simulink model "bicycle_drift_model_r_Ux_Uy"  (R2016a)
settings: Solver=VariableStepAuto  StartTime=0.0  StopTime=20  MaxStep=5e-2  RelTol=1e-3
values from neighbouring files (symbols this model uses):
  a = 0.1329    [dynamics.m]    (also in setup.m; tire_test.m = 0.11372)
  b = 0.1221    [dynamics.m]    (also in setup.m; tire_test.m = 0.14328)
  C_alpha = 120000    [dynamics.m]    (also in setup.m = 1200; tire_test.m = 197)
  initial_states_Uxy = [0.0 2 0]    [setup.m]
  Iz = 0.020899525    [dynamics.m]    (also in setup.m; tire_test.m = 0.025)
  L = 0.255    [dynamics.m]    (also in setup.m; tire_test.m = 0.257; veh_object2.m = obj_length)
  m = 2.622    [dynamics.m]    (also in setup.m; tire_test.m = 2.35)
  mu = 0.37    [dynamics.m]    (also in setup.m; tire_test.m = 1.31)
undefined symbols (not defined in the file): animation_update_interval, datetime, enable_CG_trace, enable_rearAxle_trace, plotAxisLimitMode, plotAxisLimits, save_anim_frames, vehicle_length, vehicle_width
libraries: vrlib x1, simulink x1
settings Model: Creator=Cyrus  LastModifiedBy=Cyrus

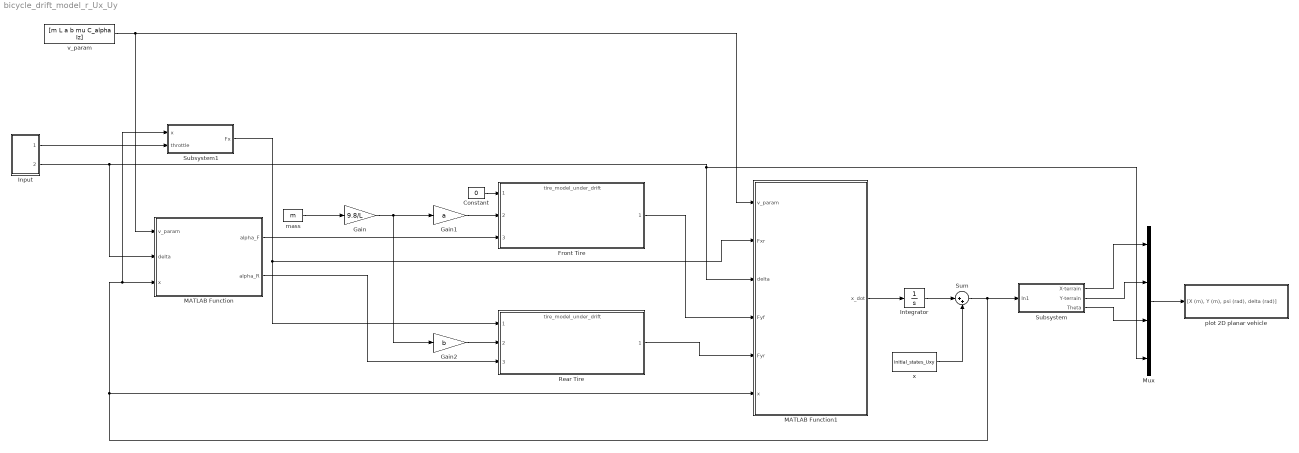
== system bicycle_drift_model_r_Ux_Uy ==
  Constant : Constant  Value=0
  Front Tire : ModelReference  ModelNameDialog=tire_model_under_drift.slx  SimulationMode=Normal  ModelReferenceVersion=1.36
  Gain : Gain  Gain=9.8/L
  Gain1 : Gain  Gain=a
  Gain2 : Gain  Gain=b
  Input : Subsystem
  Integrator : Integrator
  MATLAB Function : MATLAB Function  TreatAsAtomicUnit=on
  MATLAB Function1 : MATLAB Function  TreatAsAtomicUnit=on
  Mux : Mux
  Rear Tire : ModelReference  ModelNameDialog=tire_model_under_drift.slx  SimulationMode=Normal  ModelReferenceVersion=1.36
  Subsystem : Subsystem
  Subsystem1 : Subsystem
  Sum : Sum  Inputs=|++
  mass : Constant  Value=m
  plot 2D planar vehicle : Subsystem  mask(6DoF Animation){axisMode=plotAxisLimitMode, ax=plotAxisLimits, Ts=animation_update_interval, enable_CG_trace=enable_CG_trace, enable_rearAxle_trace=enable_rearAxle_trace, save_anim_frames=save_anim_frames, anim_frame_name_str=char(datetime('now','Format','yyyy-MM-dd_HH_mm_ss')), L=vehicle_length, W=vehicle_width}
      mask prompts: axisMode "Axis Mode (0->auto, 1->fixed, BOTH use Axes Limits below)"; ax "Axes limits [xmin xmax ymin ymax] (m):"; Ts "Time interval between updates (s):"; enable_CG_trace "Enable vehicle CG trace? (0/1)"; enable_rearAxle_trace "Enable rear axle trace? (0/1)"; save_anim_frames "Save animaton frames? (0/1)"; anim_frame_name_str "Animation sequence name (if save frames==1)"; L "Vehicle length (m)"; W "Vehicle width (m)"
      mask help:
      | Create a 2D animated view of a steering vehicle model with tires.
      |
      | Marc Compere
      | CompereM@saic.com
      | created : 22 August 2002
      | modified: 28 Dec 2015
      mask init:
      | Config.axisMode=axisMode;
      | Config.ax=ax;
      | Config.Ts=Ts;
      | Config.enable_CG_trace=enable_CG_trace;
      | Config.enable_rearAxle_trace=enable_rearAxle_trace;
      | Config.save_anim_frames=save_anim_frames;
      | Config.anim_frame_name_str=anim_frame_name_str;
      | Config.L=L;
      | Config.W=W;
      mask Help:
      | <p>This block generates a 3 dimensional display of a simulation trajectory, with the craft orientation displayed during flight</p>
      | 
      | <p>There are two inputs to this block, Position and Euler.  These inputs contain more than one signal as described below.</p>
      | 
      | <p><H4>Block Vector Input - Position</H4>
      | <ul>
      | <li>X Position</li>
      | <li>Y Position</li>
      | <li>Z Position</li>
      | </ul>
      | </p>
      | 
      | <p><H4>Block Vector Input - Euler</H4>
      |     <ul>
      |     <li>Roll Attitude</li>
      |     <li>Pitch Attitude</li>
      |     <li>Yaw Attitude</li>
      |    </ul>
      |    </p>
  v_param : Constant  Value=[m L a b mu C_alpha Iz]
  x : Constant  Value=initial_states_Uxy
  wires:
  mass/1 -> Gain/1
  Gain1/1 -> Front Tire/2
  Gain2/1 -> Rear Tire/2
  MATLAB Function/1(alpha_F) -> Front Tire/3
  MATLAB Function/2(alpha_R) -> Rear Tire/3
  Gain/1 -> Gain2/1, Gain1/1
  Sum/1 -> Subsystem1/1(x), MATLAB Function/3(x), MATLAB Function1/6(x), Subsystem/1(In1)
  MATLAB Function1/1(x_dot) -> Integrator/1
  Front Tire/1 -> MATLAB Function1/4(Fyf)
  Rear Tire/1 -> MATLAB Function1/5(Fyr)
  Constant/1 -> Front Tire/1
  Integrator/1 -> Sum/1
  x/1 -> Sum/2
  Subsystem/1(X-terrain) -> Mux/1
  Subsystem/2(Y-terrain) -> Mux/2
  Subsystem/3("Theta ") -> Mux/3
  Mux/1 -> plot 2D planar vehicle/1("[X (m), Y (m), psi (rad), delta (rad)]")
  v_param/1 -> MATLAB Function1/1(v_param), MATLAB Function/1(v_param)
  Input/2(Steering) -> MATLAB Function/2(delta), Mux/4, MATLAB Function1/3(delta)
  Input/1(Throttle) -> Subsystem1/2(throttle)
  Subsystem1/1(Fx) -> MATLAB Function1/2(Fxr), Rear Tire/1

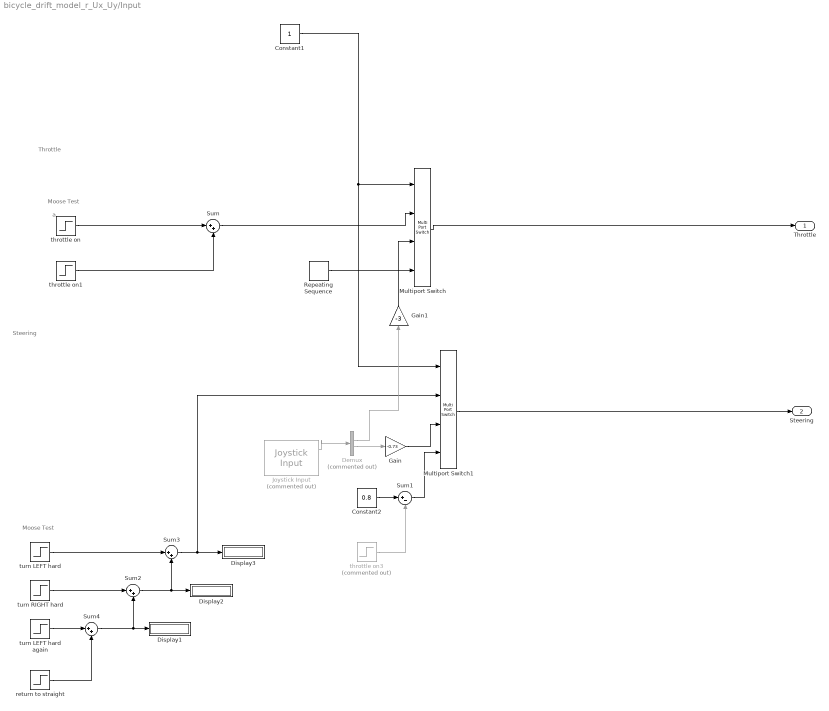
== system bicycle_drift_model_r_Ux_Uy/Input ==
  note: a
  note: Steering
  note: Throttle
  note: Moose Test
  note: Moose Test
  Constant1 : Constant
  Constant2 : Constant  Value=0.8
  Demux : Demux  Commented=on
  Display1 : Display
  Display2 : Display
  Display3 : Display
  Gain : Gain  Gain=-0.73
  Gain1 : Gain  Gain=-3  OutMin=[0.1]
  Joystick Input : vrlib/Joystick Input  Commented=on  joyid=1  adjustports=on  forcefeed=off
  Multiport Switch : MultiPortSwitch
  Multiport Switch1 : MultiPortSwitch
  Repeating Sequence : simulink/Sources/Repeating Sequence  rep_seq_t=[0 200]  rep_seq_y=[3.5 3.5]
  Sum{,2..4} (4 alike) : Sum  Inputs=|++
  Sum1 : Sum  Inputs=|+-
  return to straight : Step  Time=2.5  After=-0.83  SampleTime=0
  throttle on : Step  Time=0.2  After=3  SampleTime=0
  throttle on1 : Step  Time=3  After=-2.8  SampleTime=0
  throttle on3 : Step  Commented=on  Time=2  After=-0.8  SampleTime=0
  turn LEFT hard : Step  Time=0.3  After=0.8  SampleTime=0
  turn LEFT hard again : Step  Time=1.8  After=1.6  SampleTime=0
  turn RIGHT hard : Step  Time=0.8  After=-1.6  SampleTime=0
  Throttle : Outport
  Steering : Outport  Port=2
  wires:
  Multiport Switch1/1 -> Steering/1
  Sum/1 -> Multiport Switch/2
  throttle on1/1 -> Sum/2
  throttle on/1 -> Sum/1
  Gain/1 -> Multiport Switch1/3
  Demux/3 -> Gain/1
  Joystick Input/1 -> Demux/1
  return to straight/1 -> Sum4/2
  Sum4/1 -> Display1/1, Sum2/2
  turn RIGHT hard/1 -> Sum2/1
  turn LEFT hard/1 -> Sum3/1
  Sum3/1 -> Multiport Switch1/2, Display3/1
  Sum2/1 -> Display2/1, Sum3/2
  turn LEFT hard again/1 -> Sum4/1
  Gain1/1 -> Multiport Switch/3
  Constant1/1 -> Multiport Switch1/1, Multiport Switch/1
  Demux/2 -> Gain1/1
  Repeating Sequence/1 -> Multiport Switch/4
  Multiport Switch/1 -> Throttle/1
  Constant2/1 -> Sum1/1
  Sum1/1 -> Multiport Switch1/4
  throttle on3/1 -> Sum1/2

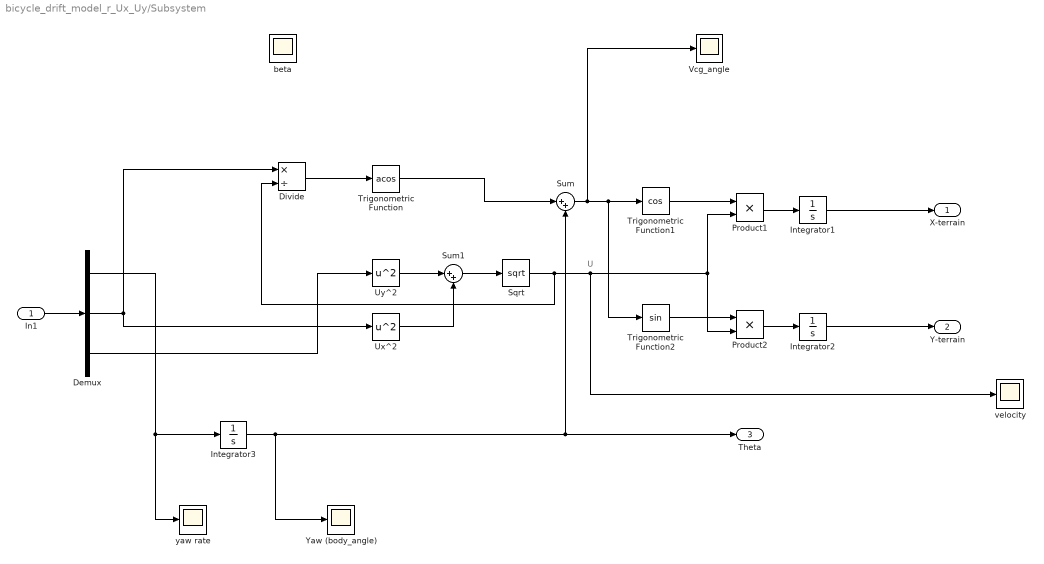
== system bicycle_drift_model_r_Ux_Uy/Subsystem ==
  note: U
  In1 : Inport
  Demux : Demux  Outputs=3
  Divide : Product  Inputs=*/
  Integrator1 : Integrator
  Integrator2 : Integrator
  Integrator3 : Integrator
  Product1 : Product
  Product2 : Product
  Sqrt : Sqrt  SaturateOnIntegerOverflow=on
  Sum : Sum  Inputs=|++
  Sum1 : Sum  Inputs=|++
  Trigonometric Function : Trigonometry  Operator=acos
  Trigonometric Function1 : Trigonometry  Operator=cos
  Trigonometric Function2 : Trigonometry
  Ux^2 : Math  Operator=square  SaturateOnIntegerOverflow=on
  Uy^2 : Math  Operator=square  SaturateOnIntegerOverflow=on
  Vcg_angle : Scope
  Yaw (body_angle) : Scope
  beta : Scope
  velocity : Scope
  yaw rate : Scope
  X-terrain : Outport
  Y-terrain : Outport  Port=2
  "Theta " : Outport  Port=3
  wires:
  In1/1 -> Demux/1
  Trigonometric Function1/1 -> Product1/1
  Trigonometric Function2/1 -> Product2/1
  Product1/1 -> Integrator1/1
  Product2/1 -> Integrator2/1
  Integrator1/1 -> X-terrain/1
  Integrator2/1 -> Y-terrain/1
  Integrator3/1 -> "Theta "/1, Sum/2, Yaw (body_angle)/1
  Sum/1 -> Vcg_angle/1, Trigonometric Function2/1, Trigonometric Function1/1
  Sqrt/1 -> Divide/2, velocity/1, Product1/2, Product2/2
  Sum1/1 -> Sqrt/1
  Uy^2/1 -> Sum1/1
  Ux^2/1 -> Sum1/2
  Divide/1 -> Trigonometric Function/1
  Trigonometric Function/1 -> Sum/1
  Demux/1 -> yaw rate/1, Integrator3/1
  Demux/2 -> Divide/1, Ux^2/1
  Demux/3 -> Uy^2/1

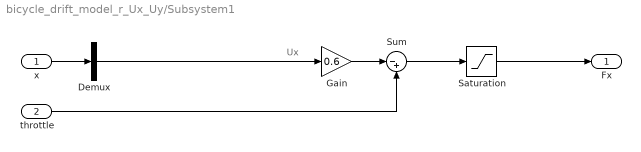
== system bicycle_drift_model_r_Ux_Uy/Subsystem1 ==
  note: Ux
  x : Inport
  throttle : Inport  Port=2
  Demux : Demux  Outputs=3
  Gain : Gain  Gain=0.6
  Saturation : Saturate  UpperLimit=mu*m*9.8*b/L  LowerLimit=-mu*m*9.8*b/L
  Sum : Sum  Inputs=|-+
  Fx : Outport
  wires:
  x/1 -> Demux/1
  Gain/1 -> Sum/1
  throttle/1 -> Sum/2
  Sum/1 -> Saturation/1
  Saturation/1 -> Fx/1
  Demux/2 -> Gain/1

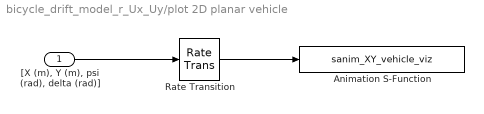
== system bicycle_drift_model_r_Ux_Uy/plot 2D planar vehicle ==
  "[X (m), Y (m), psi (rad), delta (rad)]" : Inport
  Animation S-Function : S-Function  FunctionName=sanim_XY_vehicle_viz  Parameters=Config  SFunctionDeploymentMode=off  EnableBusSupport=off
  Rate Transition : RateTransition  Integrity=off
  wires:
  "[X (m), Y (m), psi (rad), delta (rad)]"/1 -> Rate Transition/1
  Rate Transition/1 -> Animation S-Function/1

== matlab function bicycle_drift_model_r_Ux_Uy/MATLAB Function1 ==
  data: v_param input; Fxr input; delta input; Fyf input; Fyr input; x_dot output; x input
function x_dot = fcn(v_param,Fxr,delta,Fyf,Fyr,x)
%#codegen
m = v_param(1);
a = v_param(3);
b = v_param(4);
Iz = v_param(7);

r = x(1);
Ux = x(2);
Uy = x(3);

fr = 0.001*m*9.8*sign(Ux); % rolling resistance
if Ux < 0.01
    fr = 0;
end

r_dot = (a*Fyf*cos(delta)-b*Fyr)/Iz;
Ux_dot = (Fxr-Fyf*sin(delta)-fr)/m + r*Uy;
Uy_dot = (Fyf*cos(delta)+Fyr)/m - r*Ux;

x_dot = [r_dot Ux_dot Uy_dot];

== matlab function bicycle_drift_model_r_Ux_Uy/MATLAB Function ==
  data: v_param input; delta input; x input; alpha_F output; alpha_R output
function [alpha_F, alpha_R] = fcn(v_param,delta,x)
%#codegen
a = v_param(3);
b = v_param(4);

r = x(1);
Ux = x(2);
Uy = x(3);

alpha_F = atan((Uy+a*r)/Ux)-delta;
alpha_R = atan((Uy-b*r)/Ux);
